simulink model "robust"  (R2021b)
settings: Solver=VariableStepAuto  StartTime=0.0  StopTime=120  RelTol=1e-3
settings Model: Creator=16sek  LastModifiedBy=evana

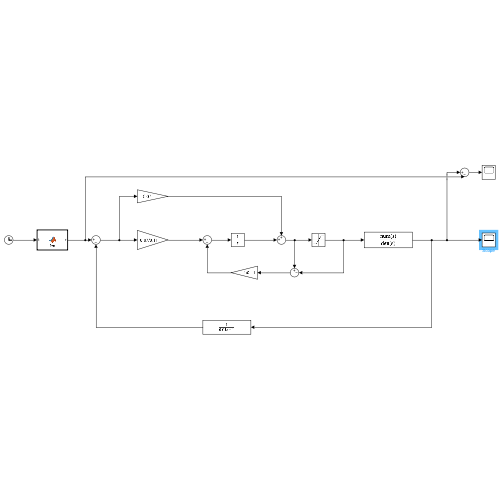
[thumbnail: Simulink's stored preview of the top-level diagram]
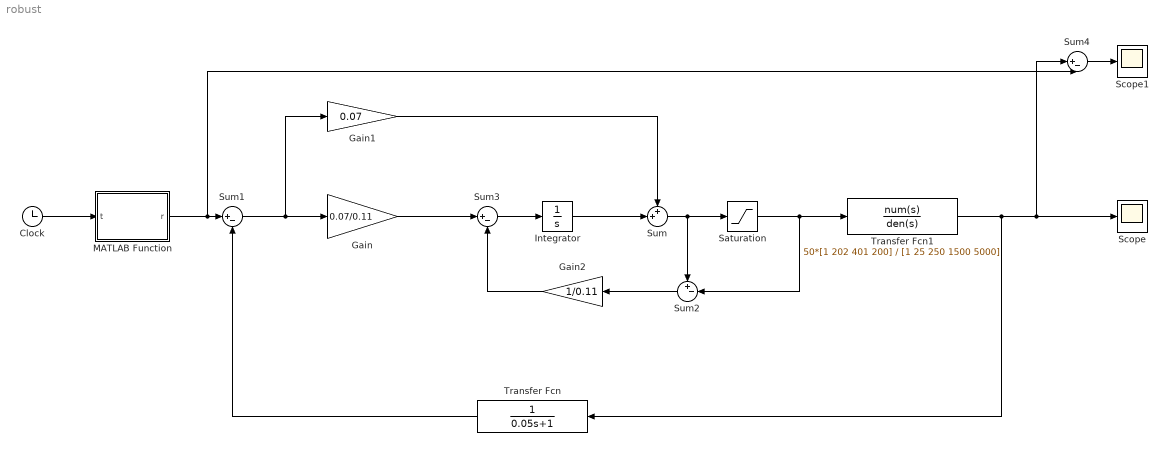
== system robust ==
  Clock : Clock
  Gain : Gain  Gain=0.07/0.11
  Gain1 : Gain  Gain=0.07
  Gain2 : Gain  Gain=1/0.11
  Integrator : Integrator
  MATLAB Function : MATLAB Function  TreatAsAtomicUnit=on
  Saturation : Saturate  UpperLimit=1  LowerLimit=-1
  Scope : Scope
      settings: Tag=y
  Scope1 : Scope
  Sum : Sum  Inputs=++|
  Sum1 : Sum  Inputs=|+-
  Sum2 : Sum  Inputs=+-|
  Sum3 : Sum  Inputs=|+-
  Sum4 : Sum  Inputs=|+-
  Transfer Fcn : TransferFcn  Denominator=[0.05 1]
  Transfer Fcn1 : TransferFcn  Numerator=50*[1 202 401 200]  Denominator=[1 25 250 1500 5000]
  wires:
  Clock/1 -> MATLAB Function/1(t)
  Sum/1 -> Sum2/1, Saturation/1
  Saturation/1 -> Transfer Fcn1/1, Sum2/2
  MATLAB Function/1(r) -> Sum4/2, Sum1/1
  Sum1/1 -> Gain/1, Gain1/1
  Integrator/1 -> Sum/2
  Gain1/1 -> Sum/1
  Sum2/1 -> Gain2/1
  Gain2/1 -> Sum3/2
  Gain/1 -> Sum3/1
  Sum3/1 -> Integrator/1
  Transfer Fcn1/1 -> Sum4/1, Scope/1, Transfer Fcn/1
  Transfer Fcn/1 -> Sum1/2
  Sum4/1 -> Scope1/1

== matlab function robust/MATLAB Function ==
  data: t input; r output
function r = fcn(t)
    if(t < 1)
        u=0;
    elseif (t<5)
        u=1;
    elseif(t<10)
        u=2;
    else
        u=-2;
    end       
r = u;
